simulink model "dynamics"  (R2024a)
settings: Solver=ode113  StartTime=0.0  StopTime=22000  RelTol=1e-3
values from neighbouring files (symbols this model uses):
  dx0 = [1; 1; 1]    [SatelliteMissionAnalysis2.m]    (also in dynamics_setup.m = [.05; .05; .05])
  Ib = [Ixx Ixy Izx ... (first row only)    [SatelliteMissionAnalysis2.m]    (also in dynamics_setup.m)
  q0 = q0/norm(q0)    [dynamics_setup.m]
  x0 = [1; 1; 1]    [SatelliteMissionAnalysis2.m]
libraries: matrix_library x2
settings Model: Creator=Zargai  LastModifiedBy=Zargai

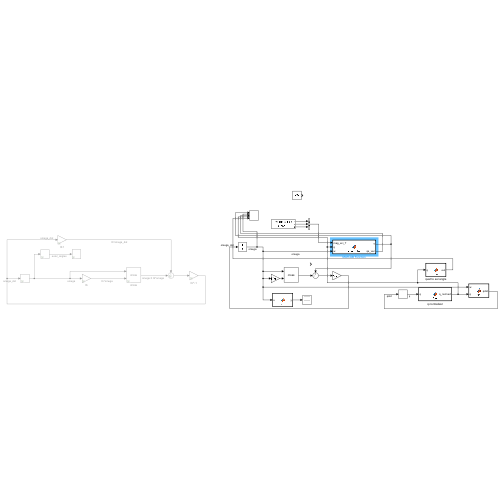
[thumbnail: Simulink's stored preview of the top-level diagram]
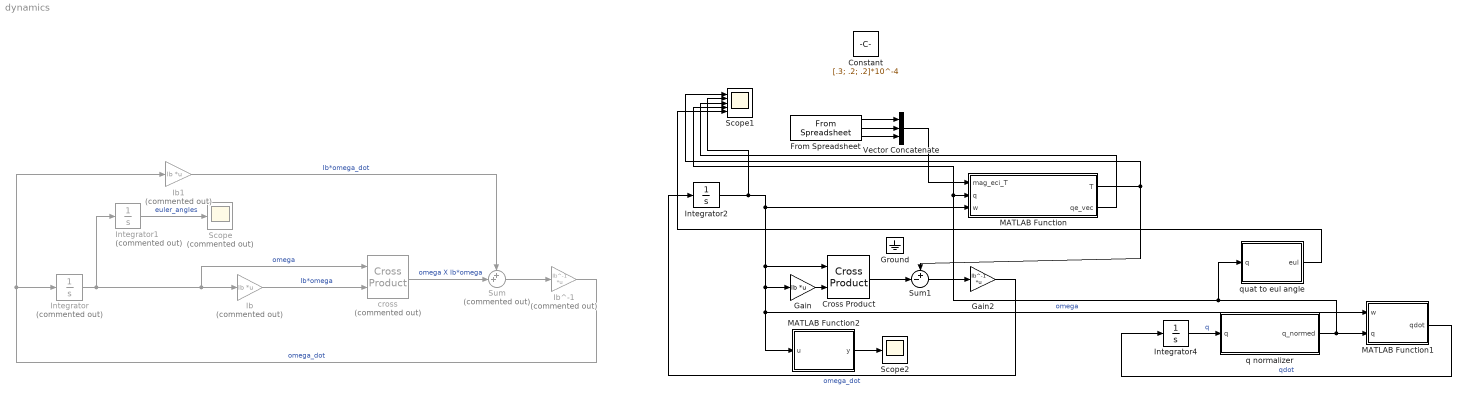
== system dynamics ==
  Constant : Constant  Value=[.3; .2; .2]*10^-4  VectorParams1D=off
  Cross Product : matrix_library/Cross Product
  From Spreadsheet : FromSpreadsheet  FileName=magdata.xlsx
  Gain : Gain  Gain=Ib  Multiplication=Matrix(K*u)
  Gain2 : Gain  Gain=Ib^-1  Multiplication=Matrix(K*u)
  Ground : Ground
  Ib : Gain  Commented=on  Gain=Ib  Multiplication=Matrix(K*u)
  Ib1 : Gain  Commented=on  Gain=Ib  Multiplication=Matrix(K*u)
  Ib^-1 : Gain  Commented=on  Gain=Ib^-1  Multiplication=Matrix(K*u)
  Integrator : Integrator  Commented=on  InitialCondition=dx0
  Integrator1 : Integrator  Commented=on  InitialCondition=x0
  Integrator2 : Integrator  InitialCondition=dx0
  Integrator4 : Integrator  InitialCondition=q0
  MATLAB Function : MATLAB Function  TreatAsAtomicUnit=on
  MATLAB Function1 : MATLAB Function  TreatAsAtomicUnit=on
  MATLAB Function2 : MATLAB Function  TreatAsAtomicUnit=on
  Scope : Scope  Commented=on
  Scope1 : Scope  NumInputPorts=5
  Scope2 : Scope
  Sum : Sum  Commented=on  Inputs=++|
  Sum1 : Sum  Inputs=+-|
  Vector Concatenate : Concatenate  NumInputs=3
  cross : matrix_library/Cross Product  Commented=on
  q normalizer : MATLAB Function  TreatAsAtomicUnit=on
  quat to eul angle : MATLAB Function  TreatAsAtomicUnit=on
  wires:
  Integrator/1 -> Ib/1, cross/1, Integrator1/1  "omega"
  Ib^-1/1 -> Ib1/1, Integrator/1  "omega_dot"
  Ib/1 -> cross/2  "Ib*omega"
  cross/1 -> Sum/2  "omega X Ib*omega"
  Ib1/1 -> Sum/1  "Ib*omega_dot"
  Sum/1 -> Ib^-1/1
  Integrator1/1 -> Scope/1  "euler_angles"
  Gain2/1 -> Integrator2/1  "omega_dot"
  Integrator2/1 -> Scope1/2, MATLAB Function2/1(u), MATLAB Function1/1(w), Gain/1, Cross Product/1, MATLAB Function/3(w)  "omega"
  Gain/1 -> Cross Product/2
  Sum1/1 -> Gain2/1
  MATLAB Function/1(T) -> Sum1/1, Scope1/1
  Cross Product/1 -> Sum1/2
  From Spreadsheet/1 -> Vector Concatenate/1
  From Spreadsheet/2 -> Vector Concatenate/2
  From Spreadsheet/3 -> Vector Concatenate/3
  MATLAB Function/2(qe_vec) -> Scope1/3
  MATLAB Function1/1(qdot) -> Integrator4/1  "qdot"
  Integrator4/1 -> q normalizer/1(q)  "q"
  q normalizer/1(q_normed) -> quat to eul angle/1(q), Scope1/4, MATLAB Function/2(q), MATLAB Function1/2(q)
  quat to eul angle/1(eul) -> Scope1/5
  Vector Concatenate/1 -> MATLAB Function/1(mag_eci_T)
  MATLAB Function2/1(y) -> Scope2/1

== matlab function dynamics/MATLAB Function1 ==
  data: w input; qdot output; q input
function qdot = fcn(w, q)

% q = wo + w1i + w2j + w3k. q = [w0 w1 w2 w3]

qdot = .5*[0 -w(1) -w(2) -w(3);
    w(1) 0 w(3) -w(2);
    w(2) -w(3) 0 w(1);
    w(3) w(2) -w(1) 0]*q;

% qdot = .5*[0 w(1) w(2) w(3);
%     -w(1) 0 w(3) -w(2);
%     -w(2) -w(3) 0 w(1);
%     -w(3) w(2) -w(1) 0]*q;

== matlab function dynamics/MATLAB Function ==
  data: mag_eci_T input; T output; q input; w input; qe_vec output
function [T, qe_vec]= controller(mag_eci_T, q, w)
% Define gains Kp and Kd
Kp = .3;
Kd = 20;

% Attitude Quat (orientation of body wrt ECI)
% As far as I understand, using the MATLAB functions as the following means
% that our attitude given by eul(1), eul(2), eul(3) is understood as a yaw
% of eul(3), then a pitch of eul(2), then a roll of eul(1).

q = quaternion(q'); % q is a column vector, q' to make it play nice with quaternion 

% Commanded Quat
qc = eul2quat([pi, 0, 0]);
qc = quaternion(qc);

% Error Quat
qe = conj(qc)*q;

% ECI to Body, take a vector in the inertial frame and write it in the body
% (rotated) frame
mag_body_T = conj(q)*quaternion([0; mag_eci_T]')*q; % q^-1*qv*q. "quaternion" function needs a row vector, not column vector

% Extract the vectors from the quat objects
[a b c d] = parts(mag_body_T);
mag_body_T = [b; c; d];

[e f g h] = parts(qe);
qe_vec = [f; g; h];

% PD Control to produce *ideal* control torque
Td = -Kp*qe_vec -Kd*w;

% Heheheh
%mag_body_T = mag_eci_T;
disp(mag_eci_T);

% "command" m
m = cross(mag_body_T, Td)/(norm(mag_body_T))^2;

% Saturate coils at .2 Am^2 (in reality, some of the directions are clipped
% at .1)

m_max = [0.2; 0.2; 0.1];
m = min(max(m, -m_max), m_max);

% Closest T in the controllable subspace to Td
T = cross(m, mag_body_T);
end

== matlab function dynamics/q normalizer ==
  data: q input; q_normed output
function q_normed = fcn(q)

q_normed = q/norm(q);

== matlab function dynamics/quat to eul angle ==
  data: q input; eul output
function eul = fcn(q)

eul = quat2eul(q');

== matlab function dynamics/MATLAB Function2 ==
  data: u input; y output
function y = fcn(u)

y = norm(u);
